simulink model "delay_pos_pos"  (R2021b)
settings: Solver=FixedStepAuto  StartTime=0.0  StopTime=30  FixedStep=Ts  MinStep=1e-5  RelTol=1e-5
undefined symbols (not defined in the file): A, A_int, B, b, Be, Bh_i, Bm, Bs, C, delayT, Dh, DiscIntNeverNeededParam, Discrete, Dm, Ds, Fc, Ff, Fip, Jh_i, Ke, Kh, Kh_i, Km, Ks, Mm, Ms, posNoiseVariance, R, Time, Ts, xe
libraries: simulink x3, ctrlSharedLib x2, cstblocks x1
settings Model: Creator=simon  LastModifiedBy=miche
settings SolverCC: AlgebraicLoopSolver=LineSearch
settings DebuggingCC: SFMachineParentedDataDiag=warning

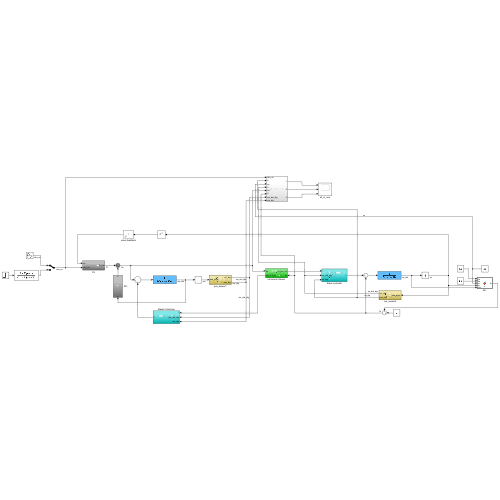
[thumbnail: Simulink's stored preview of the top-level diagram]
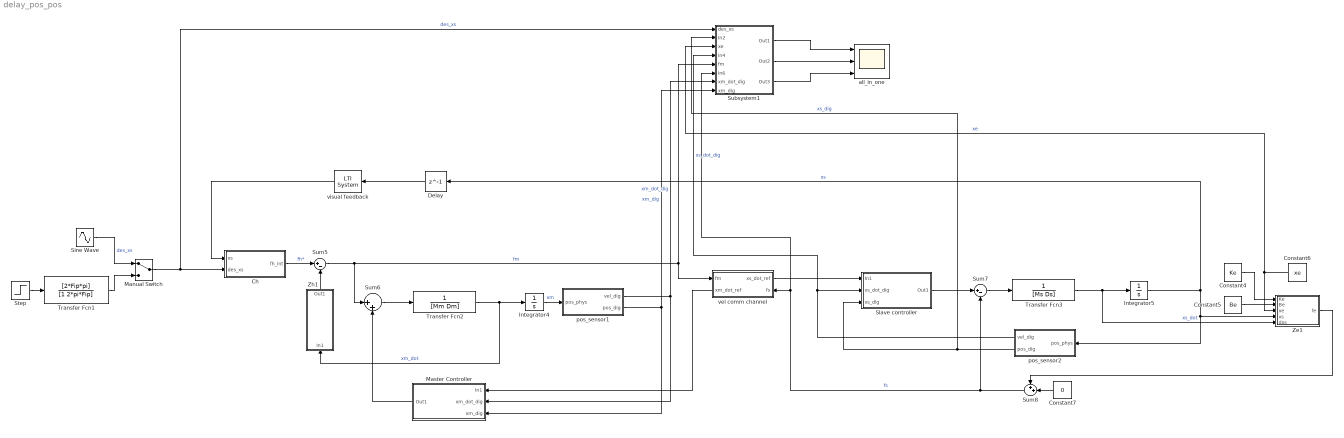
== system delay_pos_pos ==
  Ch : Subsystem
  Constant4 : Constant  Value=Ke
  Constant5 : Constant  Value=Be
  Constant6 : Constant  Value=xe
  Constant7 : Constant  Value=0
  Delay : Delay  DelayLength=1  SampleTime=Ts
  Integrator4 : Integrator
  Integrator5 : Integrator
  Manual Switch : ManualSwitch
  Master Controller : Subsystem
  Sine Wave : Sin  Amplitude=A_int  Frequency=Fc  SampleTime=0
  Slave controller : Subsystem
  Step : Step  SampleTime=0
  Subsystem1 : Subsystem
  Sum5 : Sum  Inputs=|+-
  Sum6 : Sum  Inputs=|++
  Sum7 : Sum  Inputs=|+-
  Sum8 : Sum  Inputs=++|
  Transfer Fcn1 : TransferFcn  Numerator=[2*Fip*pi]  Denominator=[1 2*pi*Fip]
  Transfer Fcn2 : TransferFcn  Denominator=[Mm Dm]
  Transfer Fcn3 : TransferFcn  Denominator=[Ms Ds]
  Ze1 : MATLAB Function  TreatAsAtomicUnit=on
  Zh1 : Subsystem
  all_in_one : Scope  NumInputPorts=3
  pos_sensor1 : Subsystem
  pos_sensor2 : Subsystem
  vel comm channel : Subsystem
      settings: PortSchema="{\"entries\":[{\"content\":{\"sides\":[{\"content\":{\"connectorIds\":[\"In1\",\"Out2\"]},\"type\":\"ConnectorPlacement.EquallySpacedRectSide\",\"uuid\":\"087ef83c-4534-4f3f-ad60-ce2423e06c57\"},{\"content\":{\"connectorIds\":[\"Out1\",\"In2\"],\"side\":\"RIGHT\"},\"type\":\"ConnectorPlacement.EquallySpacedRectSide\",\"uuid\":\"019153fa-edd0-4560-9bcd-9bc8080d4b6a\"},{\"content\":{\"connectorIds\":[],\"side\":\"TOP\"},\"type\":\"ConnectorPlacement.EquallySpacedRectSide\",\"uuid\":\"d3514247-cab7-4f3c-b49a-6c3bfe2b0cf3\"},{\"content\":{\"connectorIds\":[],\"side\":\"HIDDEN\"},\"type\":\"ConnectorPlacement.EquallySpacedRectSide\",\"uuid\":\"fe58816e-1afb-4836-94a8-7d74059b88c3\"}]},\"type\":\"ConnectorPlacement.EquallySpacedConnector\",\"uuid\":\"0c1d979d-cda7-4b3e-b96e-a73b026bb6ed\"}],\"packageUris\":[\"http://schema.mathworks.com/mf0/Connector/R2020b\"],\"version\":\"1.0\"}"
  visual feedback : cstblocks/LTI System  sys=1  IC=[]
  wires:
  Ch/1(fh_int) -> Sum5/1  "fh*"
  Sum6/1 -> Transfer Fcn2/1
  Sum5/1 -> Subsystem1/5(fm), vel comm channel/1(fm), Sum6/1  "fm"
  Zh1/1(Out1) -> Sum5/2
  Constant5/1 -> Ze1/2(Be)
  Constant6/1 -> Subsystem1/3(xe), Ze1/3(xe)  "xe"
  Integrator4/1 -> pos_sensor1/1(pos_phys)  "xm"
  Transfer Fcn2/1 -> Integrator4/1, Zh1/1(In1)  "xm_dot"
  Constant4/1 -> Ze1/1(Ke)
  pos_sensor1/1(vel_dig) -> Master Controller/2(xm_dot_dig), Subsystem1/7(xm_dot_dig)  "xm_dot_dig"
  Manual Switch/1 -> Subsystem1/1(des_xs), Ch/2(des_xs)  "des_xs"
  Delay/1 -> visual feedback/1
  visual feedback/1 -> Ch/1(xs)
  pos_sensor1/2(pos_dig) -> Master Controller/3(xm_dig), Subsystem1/8(xm_dig)  "xm_dig"
  Transfer Fcn1/1 -> Manual Switch/2
  Step/1 -> Transfer Fcn1/1
  Sine Wave/1 -> Manual Switch/1  "des_xs"
  Ze1/1(fe) -> Sum8/1
  Subsystem1/1(Out1) -> all_in_one/1
  Subsystem1/2(Out2) -> all_in_one/2
  Subsystem1/3(Out3) -> all_in_one/3
  Integrator5/1 -> Ze1/4(xs), pos_sensor2/1(pos_phys), Delay/1  "xs"
  Transfer Fcn3/1 -> Ze1/5(dxs), Integrator5/1  "xs_dot"
  Sum8/1 -> Subsystem1/6(In6), vel comm channel/2(fs), Sum7/2  "fs"
  Sum7/1 -> Transfer Fcn3/1
  Constant7/1 -> Sum8/2
  pos_sensor2/2(pos_dig) -> Slave controller/3(xs_dig), Subsystem1/2(In2)  "xs_dig"
  pos_sensor2/1(vel_dig) -> Slave controller/2(xs_dot_dig), Subsystem1/4(In4)  "xs_dot_dig"
  vel comm channel/1(xs_dot_ref) -> Slave controller/1(In1)
  Slave controller/1(Out1) -> Sum7/1
  vel comm channel/2(xm_dot_ref) -> Master Controller/1(In1)
  Master Controller/1(Out1) -> Sum6/2

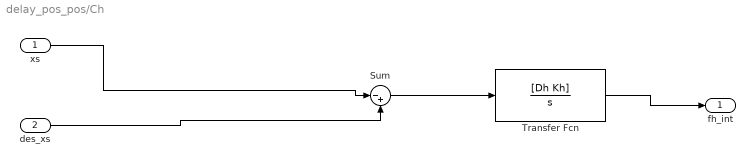
== system delay_pos_pos/Ch ==
  xs : Inport
  des_xs : Inport  Port=2
  Sum : Sum  Inputs=|-+
  Transfer Fcn : TransferFcn  Numerator=[Dh Kh]  Denominator=[1 0]
  fh_int : Outport
  wires:
  xs/1 -> Sum/1
  des_xs/1 -> Sum/2
  Sum/1 -> Transfer Fcn/1
  Transfer Fcn/1 -> fh_int/1

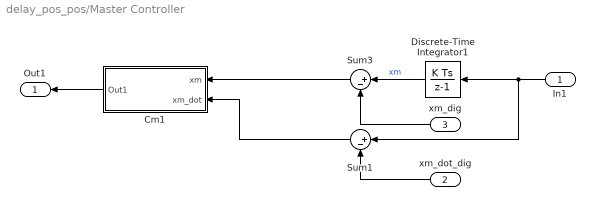
== system delay_pos_pos/Master Controller ==
  In1 : Inport
  xm_dot_dig : Inport  Port=2
  xm_dig : Inport  Port=3
  Cm1 : Subsystem
  Discrete-Time Integrator1 : DiscreteIntegrator  SampleTime=-1  ICPrevOutput=DiscIntNeverNeededParam  ICPrevScaledInput=DiscIntNeverNeededParam
  Sum1 : Sum  Inputs=|+-
  Sum3 : Sum  Inputs=|+-
  Out1 : Outport
  wires:
  In1/1 -> Discrete-Time Integrator1/1, Sum1/1
  Sum3/1 -> Cm1/1(xm)
  Sum1/1 -> Cm1/2(xm_dot)
  Discrete-Time Integrator1/1 -> Sum3/1  "xm"
  xm_dot_dig/1 -> Sum1/2
  Cm1/1(Out1) -> Out1/1
  xm_dig/1 -> Sum3/2

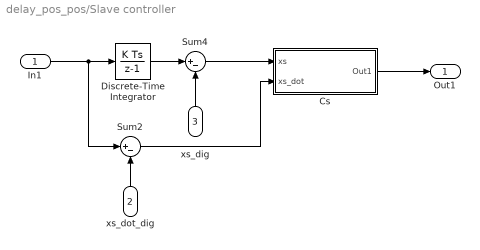
== system delay_pos_pos/Slave controller ==
  In1 : Inport
  xs_dot_dig : Inport  Port=2
  xs_dig : Inport  Port=3
  Cs : Subsystem
  Discrete-Time Integrator : DiscreteIntegrator  SampleTime=-1  ICPrevOutput=DiscIntNeverNeededParam  ICPrevScaledInput=DiscIntNeverNeededParam
  Sum2 : Sum  Inputs=|+-
  Sum4 : Sum  Inputs=|+-
  Out1 : Outport
  wires:
  In1/1 -> Sum2/1, Discrete-Time Integrator/1
  Sum2/1 -> Cs/2(xs_dot)
  xs_dot_dig/1 -> Sum2/2
  Cs/1(Out1) -> Out1/1
  xs_dig/1 -> Sum4/2
  Sum4/1 -> Cs/1(xs)
  Discrete-Time Integrator/1 -> Sum4/1

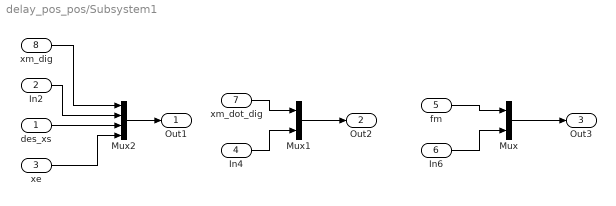
== system delay_pos_pos/Subsystem1 ==
  des_xs : Inport
  In2 : Inport  Port=2
  xe : Inport  Port=3
  In4 : Inport  Port=4
  fm : Inport  Port=5
  In6 : Inport  Port=6
  xm_dot_dig : Inport  Port=7
  xm_dig : Inport  Port=8
  Mux : Mux  Inputs=2
  Mux1 : Mux  Inputs=2
  Mux2 : Mux
  Out1 : Outport
  Out2 : Outport  Port=2
  Out3 : Outport  Port=3
  wires:
  In2/1 -> Mux2/2
  xe/1 -> Mux2/4
  Mux/1 -> Out3/1
  des_xs/1 -> Mux2/3
  Mux1/1 -> Out2/1
  xm_dot_dig/1 -> Mux1/1
  Mux2/1 -> Out1/1
  xm_dig/1 -> Mux2/1
  In6/1 -> Mux/2
  In4/1 -> Mux1/2
  fm/1 -> Mux/1

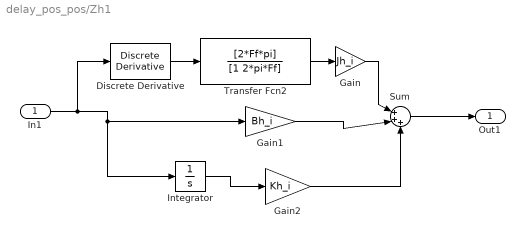
== system delay_pos_pos/Zh1 ==
  In1 : Inport
  Discrete Derivative : simulink/Discrete/Discrete Derivative  gainval=1.0  ICPrevScaledInput=0.0  OutMin=[]  OutMax=[]  OutDataType=fixdt(1, 16)  OutScaling=2^-10  DoSatur=off
  Gain : Gain  Gain=Jh_i
  Gain1 : Gain  Gain=Bh_i
  Gain2 : Gain  Gain=Kh_i
  Integrator : Integrator
  Sum : Sum  Inputs=|+++
  Transfer Fcn2 : TransferFcn  Numerator=[2*Ff*pi]  Denominator=[1 2*pi*Ff]
  Out1 : Outport
  wires:
  Integrator/1 -> Gain2/1
  In1/1 -> Integrator/1, Gain1/1, Discrete Derivative/1
  Gain/1 -> Sum/1
  Gain1/1 -> Sum/2
  Gain2/1 -> Sum/3
  Sum/1 -> Out1/1
  Transfer Fcn2/1 -> Gain/1
  Discrete Derivative/1 -> Transfer Fcn2/1

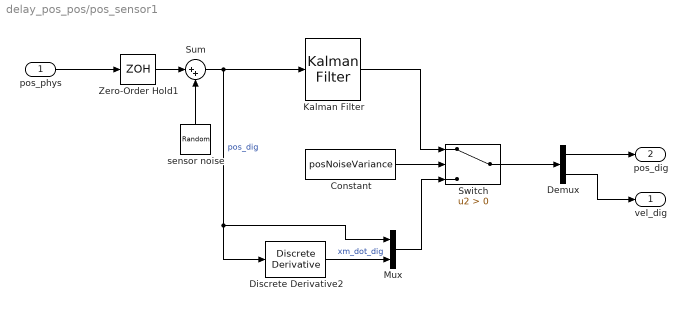
== system delay_pos_pos/pos_sensor1 ==
  pos_phys : Inport
  Constant : Constant  Value=posNoiseVariance
  Demux : Demux  Outputs=2
  Discrete Derivative2 : simulink/Discrete/Discrete Derivative  gainval=1.0  ICPrevScaledInput=0.0  OutMin=[]  OutMax=[]  OutDataType=fixdt(1, 16)  OutScaling=2^-10  DoSatur=off
  Kalman Filter : ctrlSharedLib/Kalman Filter  TimeDomain=Discrete-Time  UseCurrentEstimator=on  ModelSource=Individual A, B, C, D matrices  ModelSourceVariable=ss(0.95,1,1,0,1)  A=A  B=B  C=C  D=0  NumberOfStates=2  NumberOfInputs=1  NumberOfOutputs=1  InitialEstimateSource=Dialog  X0=0  P0=10  UseK=off  UseGH=off  NumberOfProcessNoiseInputs=1  G=1  TimeInvariantG=on  H=0  TimeInvariantH=on  Q=Q_m  TimeInvariantQ=on  R=R  TimeInvariantR=on  N=0  TimeInvariantN=on  AddInputPort=off  AddEnablePort=off  OutputEstimatedY=off  OutputP=off  Ts=Ts
  Mux : Mux  Inputs=2
  Sum : Sum  Inputs=|++
  Switch : Switch  Criteria=u2 > Threshold
  Zero-Order Hold1 : ZeroOrderHold  SampleTime=Ts
  sensor noise : RandomNumber  Variance=posNoiseVariance  SampleTime=Ts
  vel_dig : Outport
  pos_dig : Outport  Port=2
  wires:
  pos_phys/1 -> Zero-Order Hold1/1
  Zero-Order Hold1/1 -> Sum/1
  sensor noise/1 -> Sum/2
  Kalman Filter/1 -> Switch/1
  Sum/1 -> Mux/1, Discrete Derivative2/1, Kalman Filter/1  "pos_dig"
  Constant/1 -> Switch/2
  Mux/1 -> Switch/3
  Discrete Derivative2/1 -> Mux/2  "xm_dot_dig"
  Switch/1 -> Demux/1
  Demux/1 -> pos_dig/1
  Demux/2 -> vel_dig/1

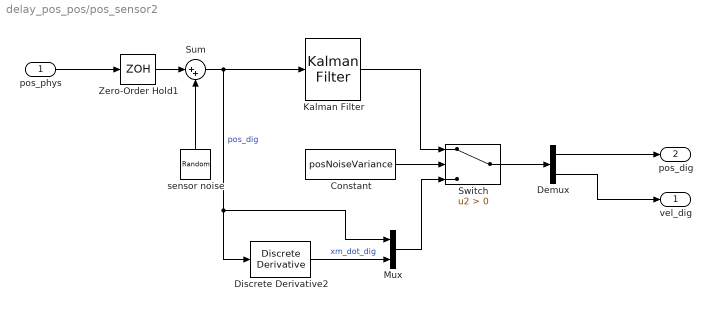
== system delay_pos_pos/pos_sensor2 ==
  pos_phys : Inport
  Constant : Constant  Value=posNoiseVariance
  Demux : Demux  Outputs=2
  Discrete Derivative2 : simulink/Discrete/Discrete Derivative  gainval=1.0  ICPrevScaledInput=0.0  OutMin=[]  OutMax=[]  OutDataType=fixdt(1, 16)  OutScaling=2^-10  DoSatur=off
  Kalman Filter : ctrlSharedLib/Kalman Filter  TimeDomain=Discrete-Time  UseCurrentEstimator=on  ModelSource=Individual A, B, C, D matrices  ModelSourceVariable=ss(0.95,1,1,0,1)  A=A  B=B  C=C  D=0  NumberOfStates=2  NumberOfInputs=1  NumberOfOutputs=1  InitialEstimateSource=Dialog  X0=0  P0=10  UseK=off  UseGH=off  NumberOfProcessNoiseInputs=1  G=1  TimeInvariantG=on  H=0  TimeInvariantH=on  Q=Q_m  TimeInvariantQ=on  R=R  TimeInvariantR=on  N=0  TimeInvariantN=on  AddInputPort=off  AddEnablePort=off  OutputEstimatedY=off  OutputP=off  Ts=Ts
  Mux : Mux  Inputs=2
  Sum : Sum  Inputs=|++
  Switch : Switch  Criteria=u2 > Threshold
  Zero-Order Hold1 : ZeroOrderHold  SampleTime=Ts
  sensor noise : RandomNumber  Variance=posNoiseVariance  SampleTime=Ts
  vel_dig : Outport
  pos_dig : Outport  Port=2
  wires:
  pos_phys/1 -> Zero-Order Hold1/1
  Zero-Order Hold1/1 -> Sum/1
  sensor noise/1 -> Sum/2
  Kalman Filter/1 -> Switch/1
  Sum/1 -> Mux/1, Discrete Derivative2/1, Kalman Filter/1  "pos_dig"
  Constant/1 -> Switch/2
  Mux/1 -> Switch/3
  Discrete Derivative2/1 -> Mux/2  "xm_dot_dig"
  Switch/1 -> Demux/1
  Demux/1 -> pos_dig/1
  Demux/2 -> vel_dig/1

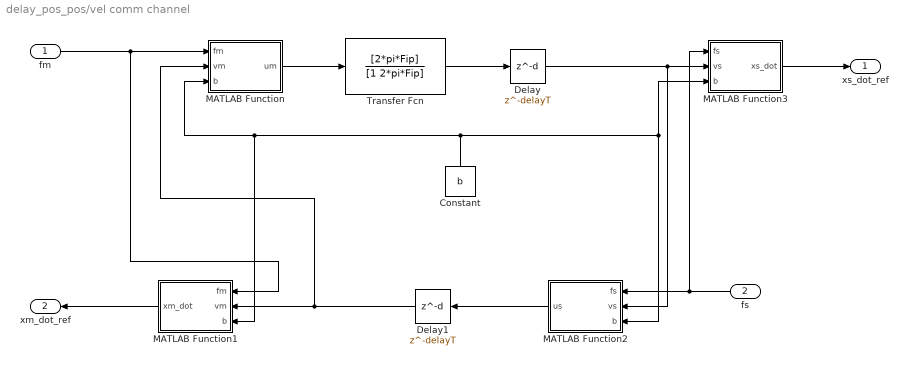
== system delay_pos_pos/vel comm channel ==
  fm : Inport
  fs : Inport  Port=2
  Constant : Constant  Value=b
  Delay : Delay  DelayLength=delayT  SampleTime=Ts
  Delay1 : Delay  DelayLength=delayT  SampleTime=Ts
  MATLAB Function : MATLAB Function  TreatAsAtomicUnit=on
  MATLAB Function1 : MATLAB Function  TreatAsAtomicUnit=on
  MATLAB Function2 : MATLAB Function  TreatAsAtomicUnit=on
  MATLAB Function3 : MATLAB Function  TreatAsAtomicUnit=on
  Transfer Fcn : TransferFcn  Numerator=[2*pi*Fip]  Denominator=[1 2*pi*Fip]
  xs_dot_ref : Outport
  xm_dot_ref : Outport  Port=2
  wires:
  Constant/1 -> MATLAB Function3/3(b), MATLAB Function2/3(b), MATLAB Function1/3(b), MATLAB Function/3(b)
  Delay/1 -> MATLAB Function2/2(vs), MATLAB Function3/2(vs)
  Delay1/1 -> MATLAB Function/2(vm), MATLAB Function1/2(vm)
  MATLAB Function/1(um) -> Transfer Fcn/1
  MATLAB Function2/1(us) -> Delay1/1
  fm/1 -> MATLAB Function1/1(fm), MATLAB Function/1(fm)
  fs/1 -> MATLAB Function2/1(fs), MATLAB Function3/1(fs)
  MATLAB Function3/1(xs_dot) -> xs_dot_ref/1
  MATLAB Function1/1(xm_dot) -> xm_dot_ref/1
  Transfer Fcn/1 -> Delay/1

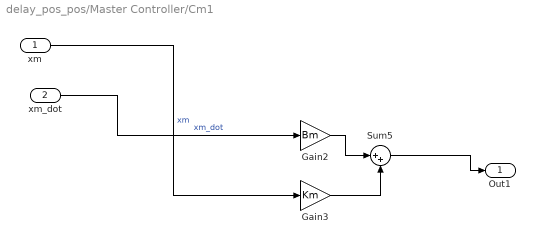
== system delay_pos_pos/Master Controller/Cm1 ==
  xm : Inport
  xm_dot : Inport  Port=2
  Gain2 : Gain  Gain=Bm
  Gain3 : Gain  Gain=Km
  Sum5 : Sum  Inputs=|++
  Out1 : Outport
  wires:
  xm/1 -> Gain3/1  "xm"
  Gain2/1 -> Sum5/1
  xm_dot/1 -> Gain2/1  "xm_dot"
  Gain3/1 -> Sum5/2
  Sum5/1 -> Out1/1

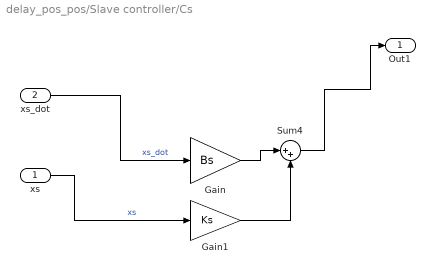
== system delay_pos_pos/Slave controller/Cs ==
  xs : Inport
  xs_dot : Inport  Port=2
  Gain : Gain  Gain=Bs
  Gain1 : Gain  Gain=Ks
  Sum4 : Sum  Inputs=|++
  Out1 : Outport
  wires:
  Gain1/1 -> Sum4/2
  Sum4/1 -> Out1/1
  xs_dot/1 -> Gain/1  "xs_dot"
  Gain/1 -> Sum4/1
  xs/1 -> Gain1/1  "xs"

== matlab function delay_pos_pos/vel comm channel/MATLAB Function ==
  data: fm input; um output; vm input; b input
function um = fcn(fm, vm, b)

um = sqrt(2/b)*fm-vm;

== matlab function delay_pos_pos/vel comm channel/MATLAB Function1 ==
  data: fm input; xm_dot output; vm input; b input
function xm_dot = fcn(fm, vm, b)

xm_dot = (1/b)*(fm-sqrt(2*b)*vm);

== matlab function delay_pos_pos/vel comm channel/MATLAB Function2 ==
  data: fs input; us output; vs input; b input
function us = fcn(fs, vs, b)

us = sqrt(2/b)*fs-vs;

== matlab function delay_pos_pos/vel comm channel/MATLAB Function3 ==
  data: fs input; xs_dot output; vs input; b input
function xs_dot = fcn(fs, vs, b)

xs_dot = -(1/b)*(fs - sqrt(2*b)*vs);

== matlab function delay_pos_pos/Ze1 ==
  data: Ke input; fe output; Be input; xe input; xs input; dxs input
function fe = env(Ke, Be, xe, xs, dxs)
    if xs > xe
        fe = Ke*(xs-xe)+Be*max(dxs, 0);
    else
        fe = 0;
    end
